simulink model "Barker_13_Correlator_f"  (R2012b)
settings: Solver=FixedStepDiscrete  StartTime=0.0  StopTime=300  RelTol=1e-3
settings Model: Creator=Carl  LastModifiedBy=Carl
settings DataIOCC: SignalLogging=off
settings OptimizationCC: BlockReduction=off  ConditionallyExecuteInputs=off  InlineParams=on
settings DebuggingCC: AlgebraicLoopMsg=error
settings HardwareCC: ProdHWDeviceType=ASIC/FPGA->ASIC/FPGA  ProdEqTarget=off

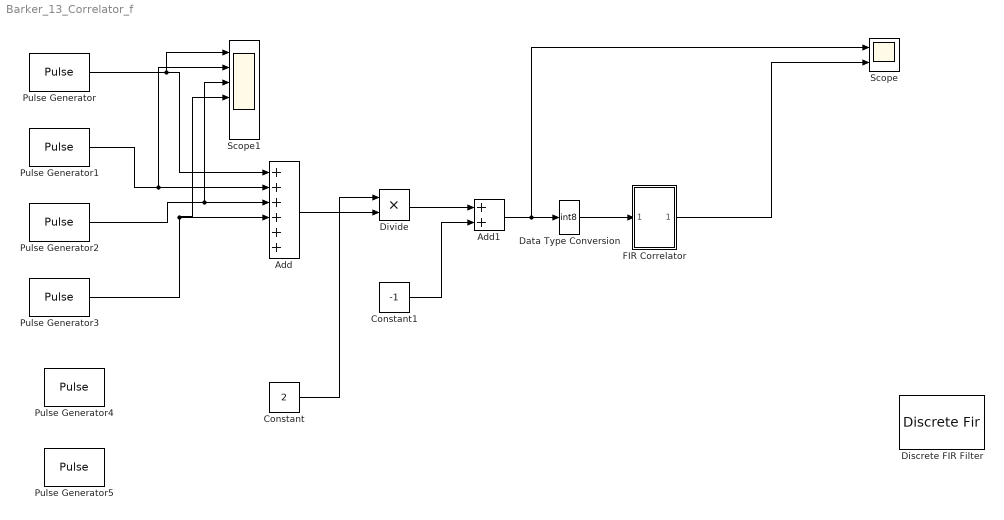
== system Barker_13_Correlator_f ==
  Add : Sum  Inputs=++++++
  Add1 : Sum
  Constant : Constant  Value=2
  Constant1 : Constant  Value=-1
  Data Type Conversion : DataTypeConversion  OutDataTypeStr=int8
  Discrete FIR Filter : DiscreteFir  FilterStructure=Direct form transposed  Coefficients=[+1 +1 +1 +1 +1 -1 -1 +1 +1 -1 +1 -1 +1]
  Divide : Product  Inputs=**
  FIR Correlator : Subsystem
  Pulse Generator : DiscretePulseGenerator  Period=100  PulseWidth=5  PhaseDelay=10
  Pulse Generator1 : DiscretePulseGenerator  Period=100  PulseWidth=2  PhaseDelay=17
  Pulse Generator2 : DiscretePulseGenerator  Period=100  PhaseDelay=20
  Pulse Generator3 : DiscretePulseGenerator  Period=100  PhaseDelay=22
  Pulse Generator4 : DiscretePulseGenerator  Amplitude=0.5  Period=100  PulseWidth=10
  Pulse Generator5 : DiscretePulseGenerator  Amplitude=0.5  Period=100  PulseWidth=100  PhaseDelay=23
  Scope : Scope  NumInputPorts=2
      settings: YMin=-5~-5  YMax=5~5
  Scope1 : Scope  NumInputPorts=6
      settings: YMin=-5~-5~-5~-5~-5~-5  YMax=5~5~5~5~5~5
  wires:
  Pulse Generator/1 -> Scope1/1, Add/1
  Pulse Generator1/1 -> Scope1/2, Add/2
  Pulse Generator2/1 -> Scope1/3, Add/3
  Pulse Generator3/1 -> Scope1/4, Add/4
  Constant/1 -> Divide/2
  Constant1/1 -> Add1/2
  Divide/1 -> Add1/1
  Add/1 -> Divide/1
  Add1/1 -> Data Type Conversion/1, Scope/1
  ? -> Scope1/5, Add/5
  ? -> Scope1/6, Add/6
  FIR Correlator/1(Out1) -> Scope/2
  Data Type Conversion/1 -> FIR Correlator/1(In1)

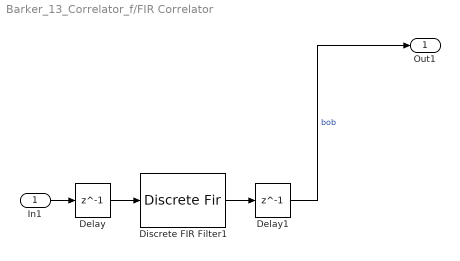
== system Barker_13_Correlator_f/FIR Correlator ==
  In1 : Inport
  Delay : Delay  DelayLength=1  InitialCondition=0
  Delay1 : Delay  DelayLength=1  InitialCondition=0
  Discrete FIR Filter1 : DiscreteFir  FilterStructure=Direct form transposed  Coefficients=[+1 -1 +1 -1 +1 +1 -1 -1 +1 +1 +1 +1 +1]  CoefDataTypeStr=fixdt(1,2,0)  ProductDataTypeStr=fixdt(1,10,0)  AccumDataTypeStr=fixdt(1,14,0)  RndMeth=Round
  Out1 : Outport
  wires:
  Discrete FIR Filter1/1 -> Delay1/1
  In1/1 -> Delay/1
  Delay/1 -> Discrete FIR Filter1/1
  Delay1/1 -> Out1/1  "bob"
